simulink model "latest_ex_9_bus_PMU"  (R2021a)
settings: Solver=ode5  StartTime=0.0  StopTime=10  RelTol=1e-3
undefined symbols (not defined in the file or in its folder): D1, Delta
libraries: spsLoadFlowBusLib x9, spsFundamentalPLLDrivenLib x6, spsPLLLib x6, spsThreePhasePISectionLineLib x6, spsThreePhaseSeriesRLCLoadLib x4, spsThreePhaseTransformerTwoWindingsLib x3, spsSynchronousMachinepuStandardLib x3, spsThreePhaseParallelRLCLoadLib x3, spsThreePhaseVIMeasurementLib x3, spsExcitationSystemLib x3, spsGenericPowerSystemStabilizerLib x3, spsHydraulicTurbineandGovernorLib x3
settings Model: Creator=z0034ktr  LastModifiedBy=yuganthadiyal
settings SolverCC: AlgebraicLoopSolver=TrustRegion  AutoInsertRateTranBlk=on
settings DebuggingCC: SFMachineParentedDataDiag=warning

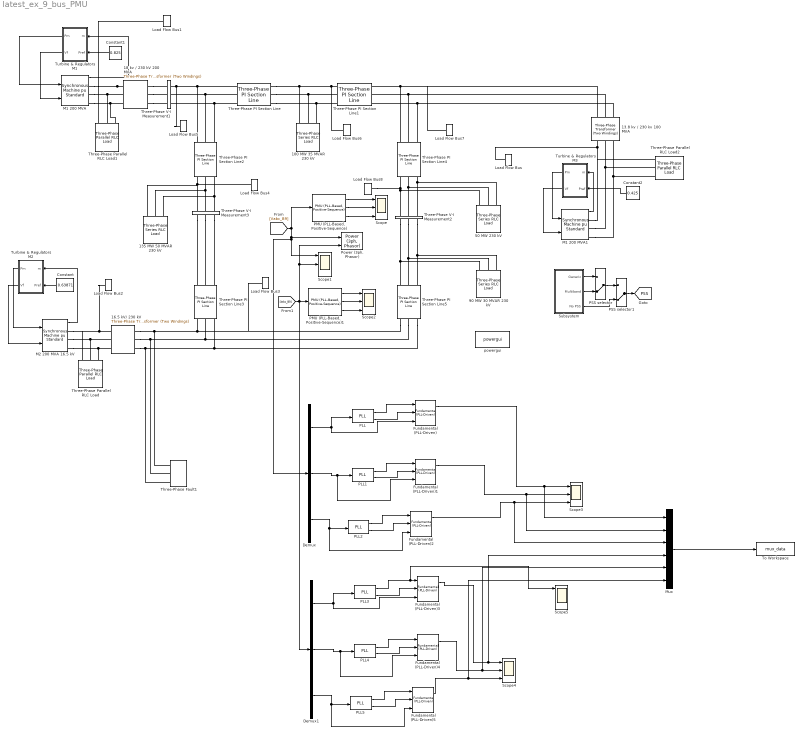
== system latest_ex_9_bus_PMU ==
  100 MW 35 MVAR 230 kV : spsThreePhaseSeriesRLCLoadLib/Three-Phase Series RLC Load  LConnTagsString=A|B|C  Configuration=Y (grounded)  NominalVoltage=(230000)*0.980041  Vabc=[1e3 1e3 1e3]  Vabcp=[1e3 1e3 1e3]  NominalFrequency=60  UnbalancedPower=off  ActivePower=100e6  InductivePower=35e6  CapacitivePower=0  Pabc=[10e3 9e3 11e3]  QLabc=[100 90 110]  QCabc=[100 90 110]  Pabcp=[10e3 9e3 11e3]  QLabcp=[100 90 110]  QCabcp=[100 90 110]  Measurements=None  LoadType=constant PQ
  13.8 kv / 230 kv 100 MVA : spsThreePhaseTransformerTwoWindingsLib/Three-Phase Transformer (Two Windings)  Winding1Connection=Delta (D1)  Winding2Connection=Yg  CoreType=Three single-phase transformers  SetSaturation=off  Hysteresis=off  DataFile='hysteresis'  SetInitialFlux=off  Measurements=None  UNITS=pu  NominalPower=[ 100e6 , 60 ]  Winding1=[ 13.8e3 , 0.002 , 0.08 ]  Winding2=[ 230e3 , 0.002 , 0.08 ]  Rm=500  Lm=500  L0=0.5  Saturation=[ 0,0 ; 0.0024,1.2 ; 1.0,1.52 ]  InitialFluxes=[ 0.8 , -0.8 , 0.7 ]  BreakLoop=off  DiscreteSolver=Trapezoidal iterative  DataType=off  TransfoNumber=1
  135 MW 50 MVAR 230 kV : spsThreePhaseSeriesRLCLoadLib/Three-Phase Series RLC Load  LConnTagsString=A|B|C  Configuration=Y (grounded)  NominalVoltage=(230000)*0.972469  Vabc=[1e3 1e3 1e3]  Vabcp=[1e3 1e3 1e3]  NominalFrequency=60  UnbalancedPower=off  ActivePower=135e6  InductivePower=50e6  CapacitivePower=0  Pabc=[10e3 9e3 11e3]  QLabc=[100 90 110]  QCabc=[100 90 110]  Pabcp=[10e3 9e3 11e3]  QLabcp=[100 90 110]  QCabcp=[100 90 110]  Measurements=None  LoadType=constant PQ
  16.5 kV/ 230 kV : spsThreePhaseTransformerTwoWindingsLib/Three-Phase Transformer (Two Windings)  Winding1Connection=Delta (D1)  Winding2Connection=Yg  CoreType=Three single-phase transformers  SetSaturation=off  Hysteresis=off  DataFile='hysteresis'  SetInitialFlux=off  Measurements=None  UNITS=pu  NominalPower=[ 200e6 , 60 ]  Winding1=[ 16.5e3 , 0.002 , 0.08 ]  Winding2=[ 230e3 , 0.002 , 0.08 ]  Rm=500  Lm=500  L0=0.5  Saturation=[ 0,0 ; 0.0024,1.2 ; 1.0,1.52 ]  InitialFluxes=[ 0.8 , -0.8 , 0.7 ]  BreakLoop=off  DiscreteSolver=Trapezoidal iterative  DataType=off  TransfoNumber=1
  18 kv / 230 kV 200 MVA : spsThreePhaseTransformerTwoWindingsLib/Three-Phase Transformer (Two Windings)  Winding1Connection=Delta (D1)  Winding2Connection=Yg  CoreType=Three single-phase transformers  SetSaturation=off  Hysteresis=off  DataFile='hysteresis'  SetInitialFlux=off  Measurements=None  UNITS=pu  NominalPower=[ 200e6 , 60 ]  Winding1=[ 18e3 , 0.002 , 0.08 ]  Winding2=[ 230e3 , 0.002 , 0.08 ]  Rm=500  Lm=500  L0=0.5  Saturation=[ 0,0 ; 0.0024,1.2 ; 1.0,1.52 ]  InitialFluxes=[ 0.8 , -0.8 , 0.7 ]  BreakLoop=off  DiscreteSolver=Trapezoidal iterative  DataType=off  TransfoNumber=1
  50 MW 230 kV : spsThreePhaseSeriesRLCLoadLib/Three-Phase Series RLC Load  LConnTagsString=A|B|C  Configuration=Y (grounded)  NominalVoltage=(230000)*0.978663  Vabc=[1e3 1e3 1e3]  Vabcp=[1e3 1e3 1e3]  NominalFrequency=60  UnbalancedPower=off  ActivePower=50e6  InductivePower=0  CapacitivePower=0  Pabc=[10e3 9e3 11e3]  QLabc=[100 90 110]  QCabc=[100 90 110]  Pabcp=[10e3 9e3 11e3]  QLabcp=[100 90 110]  QCabcp=[100 90 110]  Measurements=None  LoadType=constant PQ
  90 MW 30 MVAR 230 kV : spsThreePhaseSeriesRLCLoadLib/Three-Phase Series RLC Load  LConnTagsString=A|B|C  Configuration=Y (grounded)  NominalVoltage=(230000)*0.978663  Vabc=[1e3 1e3 1e3]  Vabcp=[1e3 1e3 1e3]  NominalFrequency=60  UnbalancedPower=off  ActivePower=90e6  InductivePower=30e6  CapacitivePower=0  Pabc=[10e3 9e3 11e3]  QLabc=[100 90 110]  QCabc=[100 90 110]  Pabcp=[10e3 9e3 11e3]  QLabcp=[100 90 110]  QCabcp=[100 90 110]  Measurements=None  LoadType=constant PQ
  Constant : Constant  Value=0.63871
  Constant1 : Constant  Value=0.825
  Constant2 : Constant  Value=0.425
  Demux : Demux  Outputs=3
  Demux1 : Demux  Outputs=3
  Fundamental (PLL-Driven){,1..5} (6 alike) : spsFundamentalPLLDrivenLib/Fundamental (PLL-Driven)  Finit=60  Fmin=45  InInit=[1, 0]  Ts=50e-5
      settings: SourceProductBaseCode=PS
  Load Flow Bus : spsLoadFlowBusLib/Load Flow Bus  LConnTagsString=a  Phases=single  Connectors=on one side  ID=BUS_3  Vbase=13.8e3  Vref=1  Vangle=0  VLF=1  VLFb=1  VLFc=1  angleLF=3.115  angleLFb=0  angleLFc=0
      settings: SourceProductBaseCode=PS
  Load Flow Bus1 : spsLoadFlowBusLib/Load Flow Bus  LConnTagsString=a  Phases=single  Connectors=on one side  ID=BUS_2  Vbase=18e3  Vref=1  Vangle=0  VLF=1  VLFb=1  VLFc=1  angleLF=3.878  angleLFb=0  angleLFc=0
      settings: SourceProductBaseCode=PS
  Load Flow Bus2 : spsLoadFlowBusLib/Load Flow Bus  LConnTagsString=a  Phases=single  Connectors=on one side  ID=BUS_1  Vbase=16.5e3  Vref=1  Vangle=0  VLF=1  VLFb=1  VLFc=1  angleLF=0  angleLFb=0  angleLFc=0
      settings: SourceProductBaseCode=PS
  Load Flow Bus3 : spsLoadFlowBusLib/Load Flow Bus  LConnTagsString=a  Phases=single  Connectors=on one side  ID=BUS_4  Vbase=230e3  Vref=1  Vangle=0  VLF=0.9805  VLFb=1  VLFc=1  angleLF=24.06  angleLFb=0  angleLFc=0
      settings: SourceProductBaseCode=PS
  Load Flow Bus4 : spsLoadFlowBusLib/Load Flow Bus  LConnTagsString=a  Phases=single  Connectors=on one side  ID=BUS_5  Vbase=230e3  Vref=1  Vangle=0  VLF=0.9725  VLFb=1  VLFc=1  angleLF=23  angleLFb=0  angleLFc=0
      settings: SourceProductBaseCode=PS
  Load Flow Bus5 : spsLoadFlowBusLib/Load Flow Bus  LConnTagsString=a  Phases=single  Connectors=on one side  ID=BUS_6  Vbase=230e3  Vref=1  Vangle=0  VLF=0.9834  VLFb=1  VLFc=1  angleLF=26.21  angleLFb=0  angleLFc=0
      settings: SourceProductBaseCode=PS
  Load Flow Bus6 : spsLoadFlowBusLib/Load Flow Bus  LConnTagsString=a  Phases=single  Connectors=on one side  ID=BUS_7  Vbase=230e3  Vref=1  Vangle=0  VLF=0.98  VLFb=1  VLFc=1  angleLF=24.57  angleLFb=0  angleLFc=0
      settings: SourceProductBaseCode=PS
  Load Flow Bus7 : spsLoadFlowBusLib/Load Flow Bus  LConnTagsString=a  Phases=single  Connectors=on one side  ID=BUS_8  Vbase=230e3  Vref=1  Vangle=0  VLF=0.988  VLFb=1  VLFc=1  angleLF=25.24  angleLFb=0  angleLFc=0
      settings: SourceProductBaseCode=PS
  Load Flow Bus8 : spsLoadFlowBusLib/Load Flow Bus  LConnTagsString=a  Phases=single  Connectors=on one side  ID=BUS_9  Vbase=230e3  Vref=1  Vangle=0  VLF=0.9787  VLFb=1  VLFc=1  angleLF=22.61  angleLFb=0  angleLFc=0
      settings: SourceProductBaseCode=PS
  M1 200 MVA : spsSynchronousMachinepuStandardLib/Synchronous Machine pu Standard  PresetModel=No  MechanicalLoad=Mechanical power Pm  ShowDetailedParameters=on  RotorType=Salient-pole  Units=per unit standard parameters  MeasurementBus=off  NominalParameters="[200E6  18000   60 ]"  Reactances1=[ 31 32 33 34 35 36 37 ]  Reactances2=[ 1.305, 0.296, 0.252, 0.474, 0.243, 0.18 ]  dAxisTimeConstants=Short-circuit  qAxisTimeConstants=Open-circuit  TimeConstants1=[]  TimeConstants2=[]  TimeConstants3=[]  TimeConstants4=[]  TimeConstants5=[ 1.01, 0.053, 0.1 ]  TimeConstants6=[]  TimeConstants7=[]  TimeConstants8=[]  StatorResistance=2.8544e-3  Mechanical="[ 3.7 0  32]"  PolePairs=32  InitialConditions=[0 -66.0372 0.836682 0.836682 0.836682 -5.70736 -125.707 114.293 1.48174]  SetSaturation=off  Saturation=[0.6404,0.7127,0.8441,0.9214,0.9956,1.082,1.19,1.316,1.457;0.7,0.7698,0.8872,0.9466,0.9969,1.046,1.1,1.151,1.201]  LoadFlowParameters=[1 950000000 0 0]  TsPowergui=0  TsBlock=-1  IterativeModel=Trapezoidal non iterative  IterativeDiscreteModel=Trapezoidal non iterative  BusType=PV  Pref=165e6  Qref=0  Qmin=-Inf  Qmax=Inf  PLF=0  QLF=0
      settings: SourceProductName=Specialized Power Systems
  M1 200 MVA1 : spsSynchronousMachinepuStandardLib/Synchronous Machine pu Standard  PresetModel=No  MechanicalLoad=Mechanical power Pm  ShowDetailedParameters=on  RotorType=Salient-pole  Units=per unit standard parameters  MeasurementBus=off  NominalParameters="[200E6  18000   60 ]"  Reactances1=[ 31 32 33 34 35 36 37 ]  Reactances2=[ 1.305, 0.296, 0.252, 0.474, 0.243, 0.18 ]  dAxisTimeConstants=Short-circuit  qAxisTimeConstants=Open-circuit  TimeConstants1=[]  TimeConstants2=[]  TimeConstants3=[]  TimeConstants4=[]  TimeConstants5=[ 1.01, 0.053, 0.1 ]  TimeConstants6=[]  TimeConstants7=[]  TimeConstants8=[]  StatorResistance=2.8544e-3  Mechanical="[ 3.7 0  32]"  PolePairs=32  InitialConditions=[0 -68.7855 0.55925 0.55925 0.55925 -4.47761 -124.478 115.522 1.04657]  SetSaturation=off  Saturation=[0.6404,0.7127,0.8441,0.9214,0.9956,1.082,1.19,1.316,1.457;0.7,0.7698,0.8872,0.9466,0.9969,1.046,1.1,1.151,1.201]  LoadFlowParameters=[1 950000000 0 0]  TsPowergui=0  TsBlock=-1  IterativeModel=Trapezoidal non iterative  IterativeDiscreteModel=Trapezoidal non iterative  BusType=PV  Pref=85e6  Qref=0  Qmin=-Inf  Qmax=Inf  PLF=0  QLF=0
      settings: SourceProductName=Specialized Power Systems
  M2 200 MVA 16.5 kV : spsSynchronousMachinepuStandardLib/Synchronous Machine pu Standard  PresetModel=No  MechanicalLoad=Mechanical power Pm  ShowDetailedParameters=on  RotorType=Salient-pole  Units=per unit standard parameters  MeasurementBus=off  NominalParameters="[200E6  16500   60 ]"  Reactances1=[ 31 32 33 34 35 36 37 ]  Reactances2=[ 1.305, 0.296, 0.252, 0.474, 0.243, 0.18 ]  dAxisTimeConstants=Short-circuit  qAxisTimeConstants=Open-circuit  TimeConstants1=[]  TimeConstants2=[]  TimeConstants3=[]  TimeConstants4=[]  TimeConstants5=[ 1.01, 0.053, 0.1 ]  TimeConstants6=[]  TimeConstants7=[]  TimeConstants8=[]  StatorResistance=2.8544e-3  Mechanical="[ 3.7 0  32]"  PolePairs=32  InitialConditions=[0 -74.1936 0.653801 0.653801 0.653801 -12.3345 -132.335 107.665 1.36624]  SetSaturation=off  Saturation=[0.6404,0.7127,0.8441,0.9214,0.9956,1.082,1.19,1.316,1.457;0.7,0.7698,0.8872,0.9466,0.9969,1.046,1.1,1.151,1.201]  LoadFlowParameters=[2 4000000000 0 0]  TsPowergui=0  TsBlock=-1  IterativeModel=Trapezoidal non iterative  IterativeDiscreteModel=Trapezoidal non iterative  BusType=swing  Pref=0  Qref=0  Qmin=-Inf  Qmax=Inf  PLF=0  QLF=0
      settings: SourceProductName=Specialized Power Systems
  Mux : Mux  Inputs=6
  PLL{,1..5} (6 alike) : spsPLLLib/PLL  Fmin=45  Par_Init=[0, 60]  ParK=[180, 3200, 1]  TcD=50e-5  MaxRateChangeFreq=12  FilterCutOffFreq=25  Ts=50e-5  AGC=on
      settings: SourceProductBaseCode=PS
  "PMU (PLL-Based, Positive-Sequence)" : spsPMUPLLBasedPositiveSequenceLib/PMU (PLL-Based, Positive-Sequence)  nominalFrequency=60  samplingRate=64  reportingFactor=1
      settings: SourceProductBaseCode=PS
  "PMU (PLL-Based, Positive-Sequence)1" : spsPMUPLLBasedPositiveSequenceLib/PMU (PLL-Based, Positive-Sequence)  nominalFrequency=60  samplingRate=64  reportingFactor=1
      settings: SourceProductBaseCode=PS
  PSS selector : ManualSwitch  CurrentSetting=0
  PSS selector1 : ManualSwitch  CurrentSetting=0
  "Power (3ph, Phasor)" : spsPower3phPhasorLib/Power (3ph, Phasor)
      settings: SourceProductBaseCode=PS
  Scope{,1..5} (6 alike) : Scope  NumInputPorts=3
  Subsystem : Subsystem
  Three-Phase PI Section Line : spsThreePhasePISectionLineLib/Three-Phase PI Section Line  LConnTagsString=a|b|c  RConnTagsString=A|B|C  Length=50  Frequency=60  Resistances=[ 0.01273 0.3864]  Inductances="[ 0.9337e-3  4.1264e-3]"  Capacitances=[12.74e-9 7.751e-9]
  Three-Phase PI Section Line1 : spsThreePhasePISectionLineLib/Three-Phase PI Section Line  LConnTagsString=a|b|c  RConnTagsString=A|B|C  Length=100  Frequency=60  Resistances=[ 0.01273 0.3864]  Inductances="[ 0.9337e-3  4.1264e-3]"  Capacitances=[12.74e-9 7.751e-9]
  Three-Phase PI Section Line2 : spsThreePhasePISectionLineLib/Three-Phase PI Section Line  LConnTagsString=a|b|c  RConnTagsString=A|B|C  Length=100  Frequency=60  Resistances=[ 0.01273 0.3864]  Inductances="[ 0.9337e-3  4.1264e-3]"  Capacitances=[12.74e-9 7.751e-9]
  Three-Phase PI Section Line3 : spsThreePhasePISectionLineLib/Three-Phase PI Section Line  LConnTagsString=a|b|c  RConnTagsString=A|B|C  Length=50  Frequency=60  Resistances=[ 0.01273 0.3864]  Inductances="[ 0.9337e-3  4.1264e-3]"  Capacitances=[12.74e-9 7.751e-9]
  Three-Phase PI Section Line4 : spsThreePhasePISectionLineLib/Three-Phase PI Section Line  LConnTagsString=a|b|c  RConnTagsString=A|B|C  Length=100  Frequency=60  Resistances=[ 0.01273 0.3864]  Inductances="[ 0.9337e-3  4.1264e-3]"  Capacitances=[12.74e-9 7.751e-9]
  Three-Phase PI Section Line5 : spsThreePhasePISectionLineLib/Three-Phase PI Section Line  LConnTagsString=a|b|c  RConnTagsString=A|B|C  Length=50  Frequency=60  Resistances=[ 0.01273 0.3864]  Inductances="[ 0.9337e-3  4.1264e-3]"  Capacitances=[12.74e-9 7.751e-9]
  Three-Phase Parallel RLC Load : spsThreePhaseParallelRLCLoadLib/Three-Phase Parallel RLC Load  LConnTagsString=A|B|C  Configuration=Y (grounded)  NominalVoltage=16.5e3  Vabc=[1e3 1e3 1e3]  Vabcp=[1e3 1e3 1e3]  NominalFrequency=60  UnbalancedPower=off  ActivePower=10e3  InductivePower=100  CapacitivePower=100  Pabc=[10e3 9e3 11e3]  QLabc=[100 90 110]  QCabc=[100 90 110]  Pabcp=[10e3 9e3 11e3]  QLabcp=[100 90 110]  QCabcp=[100 90 110]  Measurements=None  LoadType=constant Z
  Three-Phase Parallel RLC Load1 : spsThreePhaseParallelRLCLoadLib/Three-Phase Parallel RLC Load  LConnTagsString=A|B|C  Configuration=Y (grounded)  NominalVoltage=18e3  Vabc=[1e3 1e3 1e3]  Vabcp=[1e3 1e3 1e3]  NominalFrequency=60  UnbalancedPower=off  ActivePower=10e3  InductivePower=100  CapacitivePower=100  Pabc=[10e3 9e3 11e3]  QLabc=[100 90 110]  QCabc=[100 90 110]  Pabcp=[10e3 9e3 11e3]  QLabcp=[100 90 110]  QCabcp=[100 90 110]  Measurements=None  LoadType=constant Z
  Three-Phase Parallel RLC Load2 : spsThreePhaseParallelRLCLoadLib/Three-Phase Parallel RLC Load  LConnTagsString=A|B|C  Configuration=Y (grounded)  NominalVoltage=13.8e3  Vabc=[1e3 1e3 1e3]  Vabcp=[1e3 1e3 1e3]  NominalFrequency=60  UnbalancedPower=off  ActivePower=10e3  InductivePower=100  CapacitivePower=100  Pabc=[10e3 9e3 11e3]  QLabc=[100 90 110]  QCabc=[100 90 110]  Pabcp=[10e3 9e3 11e3]  QLabcp=[100 90 110]  QCabcp=[100 90 110]  Measurements=None  LoadType=constant Z
  Three-Phase V-I Measurement1 : spsThreePhaseVIMeasurementLib/Three-Phase V-I Measurement  VoltageMeasurement=phase-to-ground  SetLabelV=on  LabelV=Vabc_B6  Vpu=off  VpuLL=on  CurrentMeasurement=no  SetLabelI=off  LabelI=Iabc  Ipu=off  Pbase=100e6  Vbase=230e3  OutputType=Complex  PhasorSimulation=off  PSBequivalent=0
  Three-Phase V-I Measurement2 : spsThreePhaseVIMeasurementLib/Three-Phase V-I Measurement  VoltageMeasurement=phase-to-ground  SetLabelV=on  LabelV=Vabc_B9  Vpu=on  VpuLL=off  CurrentMeasurement=yes  SetLabelI=on  LabelI=Iabc_B9  Ipu=off  Pbase=100e6  Vbase=230e3  OutputType=Complex  PhasorSimulation=off  PSBequivalent=0
  Three-Phase V-I Measurement3 : spsThreePhaseVIMeasurementLib/Three-Phase V-I Measurement  VoltageMeasurement=phase-to-ground  SetLabelV=on  LabelV=Vabc_B1  Vpu=on  VpuLL=off  CurrentMeasurement=yes  SetLabelI=on  LabelI=Iabc_B1  Ipu=off  Pbase=100e6  Vbase=230e3  OutputType=Complex  PhasorSimulation=off  PSBequivalent=0
  Three-Phase Fault1 : spsThreePhaseFaultLib/Three-Phase Fault  InitialStates=0  FaultA=off  FaultB=on  FaultC=on  GroundFault=off  SwitchTimes=[2.5 2.6]  External=off  SwitchStatus=NaN  FaultResistance=0.001  GroundResistance=0.01  SnubberResistance=1e6  SnubberCapacitance=inf  Measurements=None
  To Workspace : ToWorkspace  VariableName=mux_data  SaveFormat=Timeseries  SampleTime=-1
  Turbine & Regulators M1 : Subsystem
  Turbine & Regulators M2 : Subsystem
  Turbine & Regulators M3 : Subsystem
  powergui : spspowerguiLib/powergui  Priority=1  SimulationMode=Discrete  SampleTime=50e-5  frequency=60  Iterations=50  frequencyindice=60  Pbase=200  ErrMax=0.0001  UnitsV=kV  UnitsW=MW  buscounter=0  FunctionMessages=off  echomessages=off  EnableUseOfTLC=off  CurrentSourceSwitches=off  DisableSnubberDevices=off  DisableRonSwitches=off  DisableVfSwitches=off  DisplayEquations=off  AutomaticDiscreteSolvers=off  SolverType=Backward Euler  Interpol=off  ExternalGateDelay=off  methode=off  Ts=100  x0status=blocks  SPID=on  SwTol=0  HookPort=off  NonlinearTolerance=1e-4  nMaxIteration=100  ContinueOnMaxIteration=off  RestoreLinks=warning  ResistiveCurrentMeasurement=off  Frange=[0:2:500]  Ylog=off  Xlog=on  ShowGrid=off  save=off  variable=ZData  structure=0  ZoomFFT=off  StartTime=0.0  cycles=1  DisplayStyle=1  fundamental=60  FreqAxis=off  MaxFrequency=1000  frequencyindicesteady=1  RmsSteady=1  display=off
  tag scope: PSS=global
  wires:
  "PMU (PLL-Based, Positive-Sequence)"/3 -> Scope/3
  "PMU (PLL-Based, Positive-Sequence)"/2 -> Scope/2
  "PMU (PLL-Based, Positive-Sequence)"/1 -> Scope/1
  M2 200 MVA 16.5 kV/1 -> Turbine & Regulators M2/1(m)
  Turbine & Regulators M2/2(Vf) -> M2 200 MVA 16.5 kV/2
  Turbine & Regulators M2/1(Pm) -> M2 200 MVA 16.5 kV/1
  Constant/1 -> Turbine & Regulators M2/2(Pref)
  PSS selector/1 -> PSS selector1/1
  Subsystem/1(Generic) -> PSS selector/1
  Subsystem/3(No PSS) -> PSS selector1/2
  Subsystem/2(Multiband) -> PSS selector/2
  PSS selector1/1 -> [PSS]
  M1 200 MVA/1 -> Turbine & Regulators M1/1(m)
  Constant1/1 -> Turbine & Regulators M1/2(Pref)
  Turbine & Regulators M1/1(Pm) -> M1 200 MVA/1
  Turbine & Regulators M1/2(Vf) -> M1 200 MVA/2
  Turbine & Regulators M3/2(Vf) -> M1 200 MVA1/2
  Turbine & Regulators M3/1(Pm) -> M1 200 MVA1/1
  M1 200 MVA1/1 -> Turbine & Regulators M3/1(m)
  Constant2/1 -> Turbine & Regulators M3/2(Pref)
  "PMU (PLL-Based, Positive-Sequence)1"/1 -> Scope2/1
  "PMU (PLL-Based, Positive-Sequence)1"/2 -> Scope2/2
  "PMU (PLL-Based, Positive-Sequence)1"/3 -> Scope2/3
  PLL/1 -> Fundamental (PLL-Driven)/1
  PLL/2 -> Fundamental (PLL-Driven)/2
  Fundamental (PLL-Driven)/1 -> Mux/1, Scope3/1
  [Vabc_B9] -> "Power (3ph, Phasor)"/1, Demux/1, Scope1/1, "PMU (PLL-Based, Positive-Sequence)"/1
  Fundamental (PLL-Driven)1/1 -> Mux/2, Scope3/2
  PLL1/2 -> Fundamental (PLL-Driven)1/2
  PLL1/1 -> Fundamental (PLL-Driven)1/1
  PLL2/1 -> Fundamental (PLL-Driven)2/1
  PLL2/2 -> Fundamental (PLL-Driven)2/2
  Fundamental (PLL-Driven)2/1 -> Mux/3, Scope3/3
  Demux/1 -> PLL/1, Fundamental (PLL-Driven)/3
  Demux/2 -> Fundamental (PLL-Driven)1/3, PLL1/1
  Demux/3 -> Fundamental (PLL-Driven)2/3, PLL2/1
  Demux1/3 -> PLL5/1, Fundamental (PLL-Driven)5/3
  Demux1/2 -> PLL4/1, Fundamental (PLL-Driven)4/3
  Demux1/1 -> Fundamental (PLL-Driven)3/3, PLL3/1
  Fundamental (PLL-Driven)5/1 -> Mux/6, Scope4/3
  PLL5/2 -> Fundamental (PLL-Driven)5/2
  PLL5/1 -> Fundamental (PLL-Driven)5/1
  PLL4/1 -> Fundamental (PLL-Driven)4/1
  PLL4/2 -> Fundamental (PLL-Driven)4/2
  Fundamental (PLL-Driven)4/1 -> Mux/5, Scope4/2
  Fundamental (PLL-Driven)3/1 -> Mux/4, Scope4/1
  PLL3/2 -> Fundamental (PLL-Driven)3/2
  PLL3/1 -> Scope5/1, Fundamental (PLL-Driven)3/1
  [Iabc_B9] -> "Power (3ph, Phasor)"/2, Scope1/2, Demux1/1, "PMU (PLL-Based, Positive-Sequence)1"/1
  Mux/1 -> To Workspace/1
  connections:
  16.5 kV/ 230 kV/RConn1 -- Three-Phase Fault1/LConn1 -- Load Flow Bus3/LConn1 -- Three-Phase PI Section Line5/RConn1 -- Three-Phase PI Section Line3/RConn1
  16.5 kV/ 230 kV/RConn2 -- Three-Phase Fault1/LConn2 -- Three-Phase PI Section Line5/RConn2 -- Three-Phase PI Section Line3/RConn2
  16.5 kV/ 230 kV/RConn3 -- Three-Phase PI Section Line5/RConn3 -- Three-Phase PI Section Line3/RConn3 -- Three-Phase Fault1/LConn3
  50 MW 230 kV/LConn1 -- Three-Phase PI Section Line4/RConn1 -- Load Flow Bus8/LConn1 -- Three-Phase V-I Measurement2/RConn1
  Three-Phase PI Section Line5/LConn3 -- Three-Phase V-I Measurement2/LConn3 -- 90 MW 30 MVAR 230 kV/LConn3
  Three-Phase PI Section Line4/LConn1 -- Load Flow Bus7/LConn1 -- 13.8 kv / 230 kv 100 MVA/RConn1 -- Three-Phase PI Section Line1/RConn1
  Three-Phase PI Section Line4/LConn2 -- 13.8 kv / 230 kv 100 MVA/RConn2 -- Three-Phase PI Section Line1/RConn2
  Three-Phase PI Section Line4/LConn3 -- 13.8 kv / 230 kv 100 MVA/RConn3 -- Three-Phase PI Section Line1/RConn3
  Three-Phase PI Section Line/RConn1 -- 100 MW 35 MVAR 230 kV/LConn1 -- Load Flow Bus6/LConn1 -- Three-Phase PI Section Line1/LConn1
  Three-Phase PI Section Line/RConn2 -- 100 MW 35 MVAR 230 kV/LConn2 -- Three-Phase PI Section Line1/LConn2
  Three-Phase PI Section Line/RConn3 -- 100 MW 35 MVAR 230 kV/LConn3 -- Three-Phase PI Section Line1/LConn3
  Load Flow Bus4/LConn1 -- Three-Phase V-I Measurement3/RConn1 -- 135 MW 50 MVAR 230 kV/LConn1 -- Three-Phase PI Section Line2/RConn1
  Three-Phase V-I Measurement3/LConn2 -- Three-Phase PI Section Line3/LConn2
  135 MW 50 MVAR 230 kV/LConn3 -- Three-Phase PI Section Line2/RConn3 -- Three-Phase V-I Measurement3/RConn3
  Three-Phase V-I Measurement1/RConn3 -- Three-Phase PI Section Line2/LConn3 -- Three-Phase PI Section Line/LConn3
  Three-Phase V-I Measurement1/RConn2 -- Three-Phase PI Section Line/LConn2 -- Three-Phase PI Section Line2/LConn2
  Three-Phase V-I Measurement1/RConn1 -- Load Flow Bus5/LConn1 -- Three-Phase PI Section Line2/LConn1 -- Three-Phase PI Section Line/LConn1
  18 kv / 230 kV 200 MVA/RConn3 -- Three-Phase V-I Measurement1/LConn3
  18 kv / 230 kV 200 MVA/RConn2 -- Three-Phase V-I Measurement1/LConn2
  18 kv / 230 kV 200 MVA/RConn1 -- Three-Phase V-I Measurement1/LConn1
  Load Flow Bus/LConn1 -- Three-Phase Parallel RLC Load2/LConn1 -- M1 200 MVA1/RConn1 -- 13.8 kv / 230 kv 100 MVA/LConn1
  M1 200 MVA1/RConn2 -- 13.8 kv / 230 kv 100 MVA/LConn2 -- Three-Phase Parallel RLC Load2/LConn2
  M1 200 MVA1/RConn3 -- Three-Phase Parallel RLC Load2/LConn3 -- 13.8 kv / 230 kv 100 MVA/LConn3
  M1 200 MVA/RConn3 -- 18 kv / 230 kV 200 MVA/LConn3 -- Three-Phase Parallel RLC Load1/LConn3
  M1 200 MVA/RConn2 -- Three-Phase Parallel RLC Load1/LConn2 -- 18 kv / 230 kV 200 MVA/LConn2
  18 kv / 230 kV 200 MVA/LConn1 -- M1 200 MVA/RConn1 -- Three-Phase Parallel RLC Load1/LConn1 -- Load Flow Bus1/LConn1
  Load Flow Bus2/LConn1 -- Three-Phase Parallel RLC Load/LConn1 -- M2 200 MVA 16.5 kV/RConn1 -- 16.5 kV/ 230 kV/LConn1
  M2 200 MVA 16.5 kV/RConn2 -- 16.5 kV/ 230 kV/LConn2 -- Three-Phase Parallel RLC Load/LConn2
  M2 200 MVA 16.5 kV/RConn3 -- 16.5 kV/ 230 kV/LConn3 -- Three-Phase Parallel RLC Load/LConn3
  50 MW 230 kV/LConn3 -- Three-Phase V-I Measurement2/RConn3 -- Three-Phase PI Section Line4/RConn3
  Three-Phase PI Section Line5/LConn2 -- Three-Phase V-I Measurement2/LConn2 -- 90 MW 30 MVAR 230 kV/LConn2
  Three-Phase PI Section Line5/LConn1 -- Three-Phase V-I Measurement2/LConn1 -- 90 MW 30 MVAR 230 kV/LConn1
  50 MW 230 kV/LConn2 -- Three-Phase V-I Measurement2/RConn2 -- Three-Phase PI Section Line4/RConn2
  Three-Phase V-I Measurement3/LConn3 -- Three-Phase PI Section Line3/LConn3
  135 MW 50 MVAR 230 kV/LConn2 -- Three-Phase PI Section Line2/RConn2 -- Three-Phase V-I Measurement3/RConn2
  Three-Phase V-I Measurement3/LConn1 -- Three-Phase PI Section Line3/LConn1

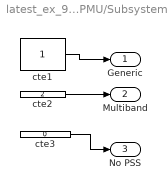
== system latest_ex_9_bus_PMU/Subsystem ==
  cte1 : Constant
  cte2 : Constant  Value=2
  cte3 : Constant  Value=0
  Generic : Outport  VectorParamsAs1DForOutWhenUnconnected=off
  Multiband : Outport  Port=2  VectorParamsAs1DForOutWhenUnconnected=off
  No PSS : Outport  Port=3  VectorParamsAs1DForOutWhenUnconnected=off
  wires:
  cte1/1 -> Generic/1
  cte2/1 -> Multiband/1
  cte3/1 -> No PSS/1

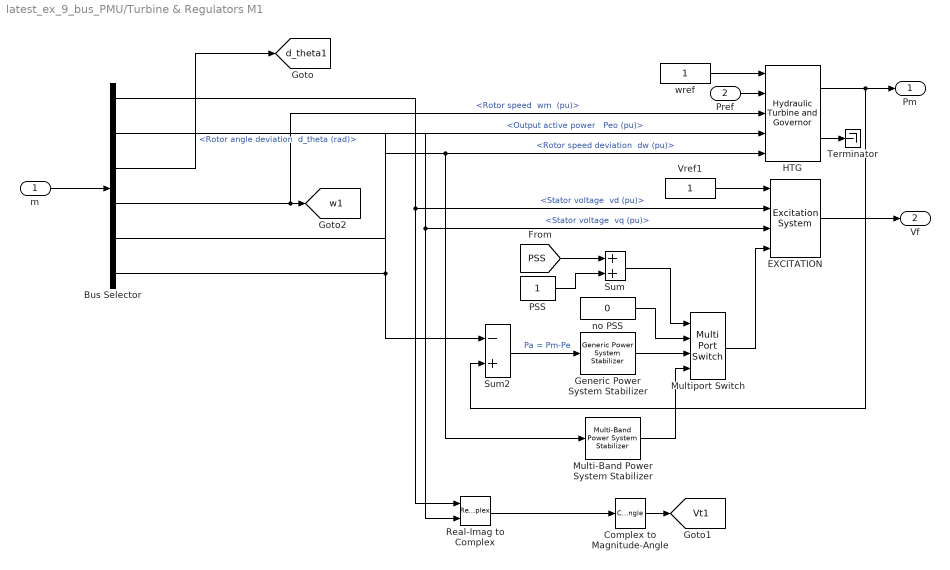
== system latest_ex_9_bus_PMU/Turbine & Regulators M1 ==
  m : Inport
  Pref : Inport  Port=2
  Bus Selector : BusSelector  OutputSignals="dq0 components.Stator voltage  vd (pu),dq0 components.Stator voltage  vq (pu),Mechanical.Rotor angle deviation  d_theta (rad),Mechanical.Rotor speed  wm  (pu),Mechanical.Rotor speed deviation  dw (pu),Output active power   Peo (pu)"
  Complex to Magnitude-Angle : ComplexToMagnitudeAngle  Output=Magnitude
  EXCITATION : spsExcitationSystemLib/Excitation System  tr=20e-3  reg=[ 200, 0.001 ]  exc=[ 1, 0 ]  tgr=[ 0, 0 ]  damp=[ 0.001, 0.1 ]  sat=[ 0, 0 ]  lim="[ 0,  7, 0 ]"  v0=[1 1.4817]
      settings: SourceProductName=Specialized Power Systems
  Generic Power System Stabilizer : spsGenericPowerSystemStabilizerLib/Generic Power System Stabilizer  Tsensor=15e-3  K=2  Twashout=0.7  Tleadlag1="[60e-3  0.5]"  Tleadlag2=[0 0]  VSlimits=[-0.15 0.15]  Vinit=0  Plot_On=off  MagdB_On=on  FreqRange=logspace(-2,2,500)
      settings: SourceProductName=Specialized Power Systems
  HTG : spsHydraulicTurbineandGovernorLib/Hydraulic Turbine and Governor  sm="[ 10/3  0.07 ]"  gate="[  0.01  0.97518  -0.1  0.1 ]"  reg="[  0.05  1.163  0.105  0  0.01  ]"  hyd="[  0  2.67  ]"  dref=0  po=0.827
      settings: SourceProductName=Specialized Power Systems
  Multi-Band Power System Stabilizer : spsMultiBandPowerSystemStabilizerLib/Multi-Band Power System Stabilizer  OperationMode=Simplified settings  Kg=1.0  GL=[0.025 5]  GI=[0.8 25]  GH=[12.0 145]  GLd=[66 66 9.4]  TcLF=[1.667 2 0 0 0 0 2 2.4 0 0 0 0 1 1]  GId=[66 66 47.6]  TcIF=[1 1 0.25 0.3 0 0 1 1 0.3 0.36 0 0 0 0]  GHd=[66 66 233]  TcHF="[0.01 0.012 0 0 0 0  0.012 0.0144 0 0 0 0 1 1]"  LIM=[.075 .15 .15 .15]  Plot_On=off  MagdB_On=off  FreqRange=logspace(-2,2,500)
      settings: SourceProductName=Specialized Power Systems
  Multiport Switch : MultiPortSwitch  SaturateOnIntegerOverflow=on
  PSS : Constant
  Real-Imag to Complex : RealImagToComplex
  Sum : Sum  SaturateOnIntegerOverflow=on
  Sum2 : Sum  Inputs=-+  InputSameDT=on  SaturateOnIntegerOverflow=on  OutDataTypeStr=Inherit: Same as first input
  Terminator : Terminator
  Vref1 : Constant
  no PSS : Constant  Value=0
  wref : Constant
  Pm : Outport  InitialOutput=0  VectorParamsAs1DForOutWhenUnconnected=off
  Vf : Outport  Port=2  InitialOutput=0  VectorParamsAs1DForOutWhenUnconnected=off
  tag scope: Vt1=global, d_theta1=global, w1=global
  wires:
  Real-Imag to Complex/1 -> Complex to Magnitude-Angle/1
  HTG/2 -> Terminator/1
  Vref1/1 -> EXCITATION/1
  m/1 -> Bus Selector/1
  Bus Selector/5 -> HTG/5, Multi-Band Power System Stabilizer/1  "<Rotor speed deviation  dw (pu)>"
  Bus Selector/4 -> HTG/3, [w1]  "<Rotor speed  wm  (pu)>"
  Pref/1 -> HTG/2
  wref/1 -> HTG/1
  HTG/1 -> Pm/1, Sum2/2
  Bus Selector/2 -> Real-Imag to Complex/2, EXCITATION/3  "<Stator voltage  vq (pu)>"
  EXCITATION/1 -> Vf/1
  Bus Selector/1 -> Real-Imag to Complex/1, EXCITATION/2  "<Stator voltage  vd (pu)>"
  Complex to Magnitude-Angle/1 -> [Vt1]
  Bus Selector/3 -> [d_theta1]  "<Rotor angle deviation  d_theta (rad)>"
  Sum2/1 -> Generic Power System Stabilizer/1  "Pa = Pm-Pe"
  Generic Power System Stabilizer/1 -> Multiport Switch/3
  Multi-Band Power System Stabilizer/1 -> Multiport Switch/4
  no PSS/1 -> Multiport Switch/2
  Multiport Switch/1 -> EXCITATION/4
  [PSS] -> Sum/1
  PSS/1 -> Sum/2
  Sum/1 -> Multiport Switch/1
  Bus Selector/6 -> HTG/4, Sum2/1  "<Output active power   Peo (pu)>"

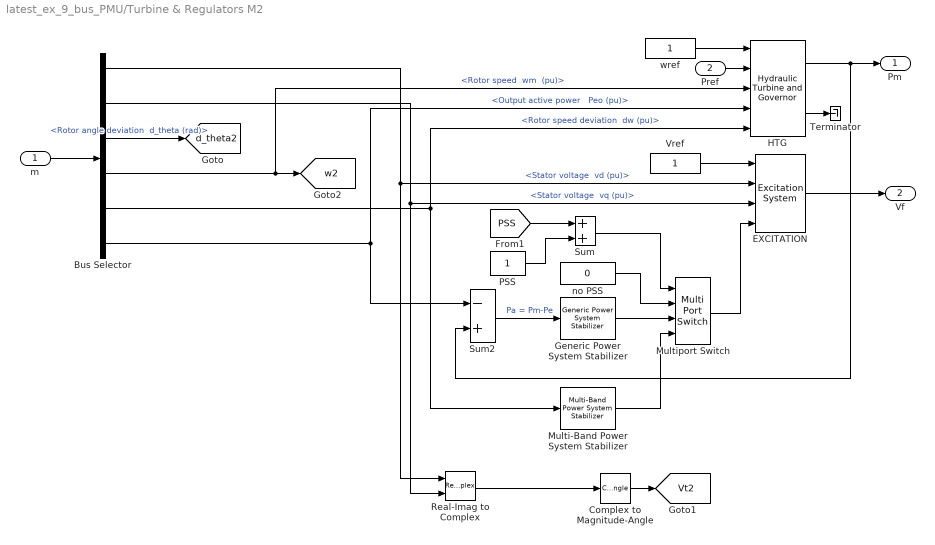
== system latest_ex_9_bus_PMU/Turbine & Regulators M2 ==
  m : Inport
  Pref : Inport  Port=2
  Bus Selector : BusSelector  OutputSignals="dq0 components.Stator voltage  vd (pu),dq0 components.Stator voltage  vq (pu),Mechanical.Rotor angle deviation  d_theta (rad),Mechanical.Rotor speed  wm  (pu),Mechanical.Rotor speed deviation  dw (pu),Output active power   Peo (pu)"
  Complex to Magnitude-Angle : ComplexToMagnitudeAngle  Output=Magnitude
  EXCITATION : spsExcitationSystemLib/Excitation System  tr=20e-3  reg=[ 200, 0.001 ]  exc=[ 1, 0 ]  tgr=[ 0, 0 ]  damp=[ 0.001, 0.1 ]  sat=[ 0, 0 ]  lim="[ 0,  7, 0 ]"  v0=[1 1.3662]
      settings: SourceProductName=Specialized Power Systems
  Generic Power System Stabilizer : spsGenericPowerSystemStabilizerLib/Generic Power System Stabilizer  Tsensor=15e-3  K=2  Twashout=0.7  Tleadlag1="[60e-3  0.5]"  Tleadlag2=[0 0]  VSlimits=[-0.15 0.15]  Vinit=0  Plot_On=off  MagdB_On=on  FreqRange=logspace(-2,2,500)
      settings: SourceProductName=Specialized Power Systems
  HTG : spsHydraulicTurbineandGovernorLib/Hydraulic Turbine and Governor  sm="[ 10/3  0.07 ]"  gate="[  0.01  0.97518  -0.1  0.1 ]"  reg="[  0.05  1.163  0.105  0  0.01  ]"  hyd="[  0  2.67  ]"  dref=0  po=0.63993
      settings: SourceProductName=Specialized Power Systems
  Multi-Band Power System Stabilizer : spsMultiBandPowerSystemStabilizerLib/Multi-Band Power System Stabilizer  OperationMode=Simplified settings  Kg=1.0  GL=[0.025 5]  GI=[0.8 25]  GH=[12.0 145]  GLd=[66 66 9.4]  TcLF=[1.667 2 0 0 0 0 2 2.4 0 0 0 0 1 1]  GId=[66 66 47.6]  TcIF=[1 1 0.25 0.3 0 0 1 1 0.3 0.36 0 0 0 0]  GHd=[66 66 233]  TcHF="[0.01 0.012 0 0 0 0  0.012 0.0144 0 0 0 0 1 1]"  LIM=[.075 .15 .15 .15]  Plot_On=off  MagdB_On=off  FreqRange=logspace(-2,2,500)
      settings: SourceProductName=Specialized Power Systems
  Multiport Switch : MultiPortSwitch  SaturateOnIntegerOverflow=on
  PSS : Constant
  Real-Imag to Complex : RealImagToComplex
  Sum : Sum  SaturateOnIntegerOverflow=on
  Sum2 : Sum  Inputs=-+  InputSameDT=on  SaturateOnIntegerOverflow=on  OutDataTypeStr=Inherit: Same as first input
  Terminator : Terminator
  Vref : Constant
  no PSS : Constant  Value=0
  wref : Constant
  Pm : Outport  InitialOutput=0  VectorParamsAs1DForOutWhenUnconnected=off
  Vf : Outport  Port=2  InitialOutput=0  VectorParamsAs1DForOutWhenUnconnected=off
  tag scope: Vt2=global, d_theta2=global, w2=global
  wires:
  PSS/1 -> Sum/2
  [PSS] -> Sum/1
  Real-Imag to Complex/1 -> Complex to Magnitude-Angle/1
  HTG/2 -> Terminator/1
  Vref/1 -> EXCITATION/1
  m/1 -> Bus Selector/1
  Bus Selector/5 -> HTG/5, Multi-Band Power System Stabilizer/1  "<Rotor speed deviation  dw (pu)>"
  Bus Selector/6 -> Sum2/1, HTG/4  "<Output active power   Peo (pu)>"
  Bus Selector/4 -> [w2], HTG/3  "<Rotor speed  wm  (pu)>"
  Pref/1 -> HTG/2
  wref/1 -> HTG/1
  HTG/1 -> Pm/1, Sum2/2
  Bus Selector/2 -> Real-Imag to Complex/2, EXCITATION/3  "<Stator voltage  vq (pu)>"
  EXCITATION/1 -> Vf/1
  Bus Selector/1 -> Real-Imag to Complex/1, EXCITATION/2  "<Stator voltage  vd (pu)>"
  Complex to Magnitude-Angle/1 -> [Vt2]
  Bus Selector/3 -> [d_theta2]  "<Rotor angle deviation  d_theta (rad)>"
  Sum2/1 -> Generic Power System Stabilizer/1  "Pa = Pm-Pe"
  Generic Power System Stabilizer/1 -> Multiport Switch/3
  Multi-Band Power System Stabilizer/1 -> Multiport Switch/4
  no PSS/1 -> Multiport Switch/2
  Sum/1 -> Multiport Switch/1
  Multiport Switch/1 -> EXCITATION/4

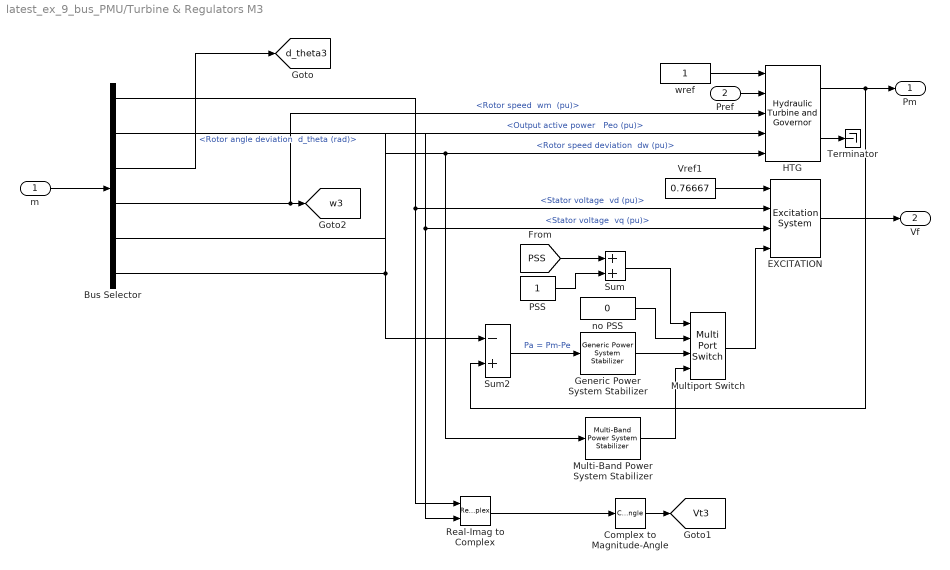
== system latest_ex_9_bus_PMU/Turbine & Regulators M3 ==
  m : Inport
  Pref : Inport  Port=2
  Bus Selector : BusSelector  OutputSignals="dq0 components.Stator voltage  vd (pu),dq0 components.Stator voltage  vq (pu),Mechanical.Rotor angle deviation  d_theta (rad),Mechanical.Rotor speed  wm  (pu),Mechanical.Rotor speed deviation  dw (pu),Output active power   Peo (pu)"
  Complex to Magnitude-Angle : ComplexToMagnitudeAngle  Output=Magnitude
  EXCITATION : spsExcitationSystemLib/Excitation System  tr=20e-3  reg=[ 200, 0.001 ]  exc=[ 1, 0 ]  tgr=[ 0, 0 ]  damp=[ 0.001, 0.1 ]  sat=[ 0, 0 ]  lim="[ 0,  7, 0 ]"  v0=[0.76667 1.0466]
      settings: SourceProductName=Specialized Power Systems
  Generic Power System Stabilizer : spsGenericPowerSystemStabilizerLib/Generic Power System Stabilizer  Tsensor=15e-3  K=2  Twashout=0.7  Tleadlag1="[60e-3  0.5]"  Tleadlag2=[0 0]  VSlimits=[-0.15 0.15]  Vinit=0  Plot_On=off  MagdB_On=on  FreqRange=logspace(-2,2,500)
      settings: SourceProductName=Specialized Power Systems
  HTG : spsHydraulicTurbineandGovernorLib/Hydraulic Turbine and Governor  sm="[ 10/3  0.07 ]"  gate="[  0.01  0.97518  -0.1  0.1 ]"  reg="[  0.05  1.163  0.105  0  0.01  ]"  hyd="[  0  2.67  ]"  dref=0  po=0.42589
      settings: SourceProductName=Specialized Power Systems
  Multi-Band Power System Stabilizer : spsMultiBandPowerSystemStabilizerLib/Multi-Band Power System Stabilizer  OperationMode=Simplified settings  Kg=1.0  GL=[0.025 5]  GI=[0.8 25]  GH=[12.0 145]  GLd=[66 66 9.4]  TcLF=[1.667 2 0 0 0 0 2 2.4 0 0 0 0 1 1]  GId=[66 66 47.6]  TcIF=[1 1 0.25 0.3 0 0 1 1 0.3 0.36 0 0 0 0]  GHd=[66 66 233]  TcHF="[0.01 0.012 0 0 0 0  0.012 0.0144 0 0 0 0 1 1]"  LIM=[.075 .15 .15 .15]  Plot_On=off  MagdB_On=off  FreqRange=logspace(-2,2,500)
      settings: SourceProductName=Specialized Power Systems
  Multiport Switch : MultiPortSwitch  SaturateOnIntegerOverflow=on
  PSS : Constant
  Real-Imag to Complex : RealImagToComplex
  Sum : Sum  SaturateOnIntegerOverflow=on
  Sum2 : Sum  Inputs=-+  InputSameDT=on  SaturateOnIntegerOverflow=on  OutDataTypeStr=Inherit: Same as first input
  Terminator : Terminator
  Vref1 : Constant  Value=0.76667
  no PSS : Constant  Value=0
  wref : Constant
  Pm : Outport  InitialOutput=0  VectorParamsAs1DForOutWhenUnconnected=off
  Vf : Outport  Port=2  InitialOutput=0  VectorParamsAs1DForOutWhenUnconnected=off
  tag scope: Vt3=global, d_theta3=global, w3=global
  wires:
  Real-Imag to Complex/1 -> Complex to Magnitude-Angle/1
  HTG/2 -> Terminator/1
  Vref1/1 -> EXCITATION/1
  m/1 -> Bus Selector/1
  Bus Selector/5 -> HTG/5, Multi-Band Power System Stabilizer/1  "<Rotor speed deviation  dw (pu)>"
  Bus Selector/4 -> HTG/3, [w3]  "<Rotor speed  wm  (pu)>"
  Pref/1 -> HTG/2
  wref/1 -> HTG/1
  HTG/1 -> Pm/1, Sum2/2
  Bus Selector/2 -> Real-Imag to Complex/2, EXCITATION/3  "<Stator voltage  vq (pu)>"
  EXCITATION/1 -> Vf/1
  Bus Selector/1 -> Real-Imag to Complex/1, EXCITATION/2  "<Stator voltage  vd (pu)>"
  Complex to Magnitude-Angle/1 -> [Vt3]
  Bus Selector/3 -> [d_theta3]  "<Rotor angle deviation  d_theta (rad)>"
  Sum2/1 -> Generic Power System Stabilizer/1  "Pa = Pm-Pe"
  Generic Power System Stabilizer/1 -> Multiport Switch/3
  Multi-Band Power System Stabilizer/1 -> Multiport Switch/4
  no PSS/1 -> Multiport Switch/2
  Multiport Switch/1 -> EXCITATION/4
  [PSS] -> Sum/1
  PSS/1 -> Sum/2
  Sum/1 -> Multiport Switch/1
  Bus Selector/6 -> HTG/4, Sum2/1  "<Output active power   Peo (pu)>"
